simulink model "simulation"  (R2015a)
settings: Solver=ode45  StartTime=0.0  StopTime=10.0  RelTol=1e-3
libraries: powerlib x63
settings Model: Creator=Syed_Sharjeel  LastModifiedBy=Syed_Sharjeel

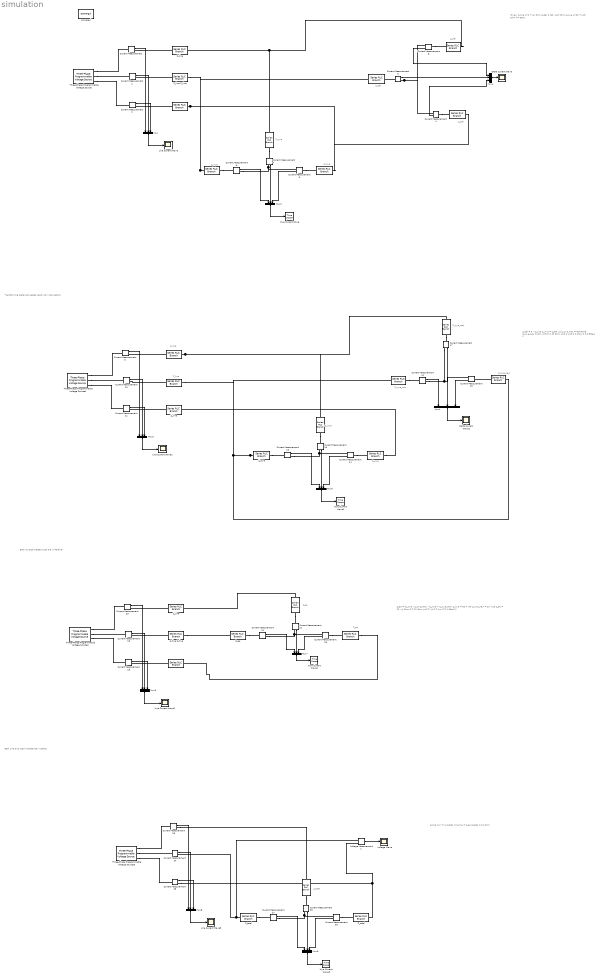
== system simulation ==
  note: Given:
      | Z_line = (2 + j4) Ohm
      | Z_del = (60 - j45) Ohm
      | Z_wye = (30 + j40) Ohm
      | f = 60Hz
  note: Z_total
  note: Z_eq
  note: Z_eq
  note: Z_line
  note: Z_line
  note: Z_wye
  note: Z_wye
  note: Z_wye
  note: Z_del
  note: Z_del
  note: Z_del
  note: Z_wye_new
  note: Z_wye_new
  note: Z_wye_new
  note: Z_wye
  note: Z_wye
  note: Z_line = 2 + j4
      | Z_total = Z_line + Z_eq
      | Z_total = 24 Ohm
  note: Both Line and Load Impedance in Series
  note: Z_eq = (Z_wye * Z_wye_new) / (Z_wye + Z_wye_new)
      | Z_wye = 30 + j40
      | Z_wye_new = 20 - j15
      | Z_eq = 22 - j4 Ohm
      | R = 22 Ohm
      | -jwC = -j4
      | C = 4/w
      | C = 1.06e-2 F
  note: Both Wye-Connected Load are in Parallel
  note: Z_del = 3 * Z_wye
      | Z_wye = Z_del / 3
      | Z_wye_new = (60-j45)/3
      | Z_wye_new = (20 - j15)
      | R = 20 Ohm
      | -jwC = -j15
      | C = 15/w
      | C = 3.98e-2 F
  note: Transforming Delta Connected Load into Y-Connection
   {,,,,} (5 alike) : powerlib/Elements/Series RLC Branch  LConnTagsString=__new0  RConnTagsString=__new0  BranchType=RL  Resistance=40  Inductance=0.66  SetiL0=off  InitialCurrent=0  Capacitance=1e-6  Setx0=off  InitialVoltage=0  Measurements=None
  " " : powerlib/Elements/Series RLC Branch  LConnTagsString=__new0  RConnTagsString=__new0  BranchType=RC  Resistance=60  Inductance=1e-3  SetiL0=off  InitialCurrent=0  Capacitance=3.703e-4  Setx0=off  InitialVoltage=0  Measurements=None
  " " : powerlib/Elements/Series RLC Branch  LConnTagsString=__new0  RConnTagsString=__new0  BranchType=RC  Resistance=20  Inductance=1e-3  SetiL0=off  InitialCurrent=0  Capacitance=3.98e-2  Setx0=off  InitialVoltage=0  Measurements=None
  " " : powerlib/Elements/Series RLC Branch  LConnTagsString=__new0  RConnTagsString=__new0  BranchType=RC  Resistance=60  Inductance=1e-3  SetiL0=off  InitialCurrent=0  Capacitance=3.703e-4  Setx0=off  InitialVoltage=0  Measurements=None
  " " : powerlib/Elements/Series RLC Branch  LConnTagsString=__new0  RConnTagsString=__new0  BranchType=RC  Resistance=20  Inductance=1e-3  SetiL0=off  InitialCurrent=0  Capacitance=3.98e-2  Setx0=off  InitialVoltage=0  Measurements=None
  " " : powerlib/Elements/Series RLC Branch  LConnTagsString=__new0  RConnTagsString=__new0  BranchType=RC  Resistance=20  Inductance=1e-3  SetiL0=off  InitialCurrent=0  Capacitance=3.98e-2  Setx0=off  InitialVoltage=0  Measurements=None
  " " : powerlib/Elements/Series RLC Branch  LConnTagsString=__new0  RConnTagsString=__new0  BranchType=RC  Resistance=60  Inductance=1e-3  SetiL0=off  InitialCurrent=0  Capacitance=3.703e-4  Setx0=off  InitialVoltage=0  Measurements=None
  " " : powerlib/Elements/Series RLC Branch  LConnTagsString=__new0  RConnTagsString=__new0  BranchType=R  Resistance=24  Inductance=0.66  SetiL0=off  InitialCurrent=0  Capacitance=1.06e-2  Setx0=off  InitialVoltage=0  Measurements=None
   {,,,} (4 alike) : powerlib/Elements/Series RLC Branch  LConnTagsString=__new0  RConnTagsString=__new0  BranchType=RL  Resistance=2  Inductance=0.066  SetiL0=off  InitialCurrent=0  Capacitance=1e-6  Setx0=off  InitialVoltage=0  Measurements=None
  " " : powerlib/Elements/Series RLC Branch  LConnTagsString=__new0  RConnTagsString=__new0  BranchType=RC  Resistance=20  Inductance=0.66  SetiL0=off  InitialCurrent=0  Capacitance=1.06e-2  Setx0=off  InitialVoltage=0  Measurements=None
  " " : powerlib/Elements/Series RLC Branch  LConnTagsString=__new0  RConnTagsString=__new0  BranchType=RC  Resistance=20  Inductance=0.66  SetiL0=off  InitialCurrent=0  Capacitance=1.06e-2  Setx0=off  InitialVoltage=0  Measurements=None
  " Z_eq " : powerlib/Elements/Series RLC Branch  LConnTagsString=__new0  RConnTagsString=__new0  BranchType=RC  Resistance=20  Inductance=0.66  SetiL0=off  InitialCurrent=0  Capacitance=1.06e-2  Setx0=off  InitialVoltage=0  Measurements=None
  " Z_line Z_line " : powerlib/Elements/Series RLC Branch  LConnTagsString=__new0  RConnTagsString=__new0  BranchType=RL  Resistance=2  Inductance=0.066  SetiL0=off  InitialCurrent=0  Capacitance=1e-6  Setx0=off  InitialVoltage=0  Measurements=None
  Current Measurement{,1..29} (30 alike) : powerlib/Measurements/Current Measurement  PhasorSimulation=off  OutputType=Complex  PSBequivalent=0
  Delta Current Wave : Scope
      settings: TimeRange=0.05  YMin=-0.09  YMax=0.12
  Delta Current Wave1 : Scope
      settings: TimeRange=0.05  YMin=-0.09  YMax=0.12  SaveName=ScopeData2
  Line Current Wave{,1..3} (4 alike) : Scope
      Line Current Wave settings: YMin=-0.025  YMax=0.025  SaveName=ScopeData4
      Line Current Wave1 settings: YMin=-0.025  YMax=0.025  SaveName=ScopeData3
      Line Current Wave2 settings: YMin=-0.025  YMax=0.025  SaveName=ScopeData5
      Line Current Wave3 settings: YMin=-0.025  YMax=0.025  SaveName=ScopeData7
  Mux{,1..9} (10 alike) : Mux  Inputs=3
  Three-Phase Programmable Voltage Source{,1..3} (4 alike) : powerlib/Electrical Sources/Three-Phase Programmable Voltage Source  PositiveSequence="[207.85  0 60]"  VariationEntity=None  VariationType=Table of time-amplitude pairs  VariationTypeAlt=Step  VariationStep=0.5  VariationRate=10  VariationMagnitude=0.3  VariationFrequency=2  VariationTiming=[1 2]  VariationPhaseA=off  Amplitudes=[1 0.8 1.2 1.0]  TimeValues=[0 0.1 0.15 0.2]  HarmonicGeneration=off  HarmonicA=[3 0.2 -25 0]  HarmonicB=[2 0.15 35 2]  Timing="[0.05  3]"  BusType=swing  Pref=0  Qref=0  Qmin=-inf  Qmax=inf
  Voltage Measurement1 : powerlib/Measurements/Voltage Measurement  PhasorSimulation=off  OutputType=Complex  PSBequivalent=0
  Voltage Wave : Scope
      settings: TimeRange=0.05  YMin=-300  YMax=300  SaveName=ScopeData11
  Wye Current Wave{,1..3} (4 alike) : TimeScope
  "Z_line " : powerlib/Elements/Series RLC Branch  LConnTagsString=__new0  RConnTagsString=__new0  BranchType=RL  Resistance=2  Inductance=0.066  SetiL0=off  InitialCurrent=0  Capacitance=1e-6  Setx0=off  InitialVoltage=0  Measurements=None
  "Z_line Z_line " : powerlib/Elements/Series RLC Branch  LConnTagsString=__new0  RConnTagsString=__new0  BranchType=RL  Resistance=2  Inductance=0.066  SetiL0=off  InitialCurrent=0  Capacitance=1e-6  Setx0=off  InitialVoltage=0  Measurements=None
  "Z_line " : powerlib/Elements/Series RLC Branch  LConnTagsString=__new0  RConnTagsString=__new0  BranchType=RL  Resistance=2  Inductance=0.066  SetiL0=off  InitialCurrent=0  Capacitance=1e-6  Setx0=off  InitialVoltage=0  Measurements=None
  "Z_line " : powerlib/Elements/Series RLC Branch  LConnTagsString=__new0  RConnTagsString=__new0  BranchType=RL  Resistance=2  Inductance=0.066  SetiL0=off  InitialCurrent=0  Capacitance=1e-6  Setx0=off  InitialVoltage=0  Measurements=None
  "Z_total " : powerlib/Elements/Series RLC Branch  LConnTagsString=__new0  RConnTagsString=__new0  BranchType=R  Resistance=24  Inductance=0.66  SetiL0=off  InitialCurrent=0  Capacitance=1.06e-2  Setx0=off  InitialVoltage=0  Measurements=None
  "Z_total " : powerlib/Elements/Series RLC Branch  LConnTagsString=__new0  RConnTagsString=__new0  BranchType=R  Resistance=24  Inductance=0.66  SetiL0=off  InitialCurrent=0  Capacitance=1.06e-2  Setx0=off  InitialVoltage=0  Measurements=None
  Z_wye : powerlib/Elements/Series RLC Branch  LConnTagsString=__new0  RConnTagsString=__new0  BranchType=RL  Resistance=40  Inductance=0.66  SetiL0=off  InitialCurrent=0  Capacitance=1e-6  Setx0=off  InitialVoltage=0  Measurements=None
  powergui : powerlib/powergui  Priority=1  SimulationMode=Discrete  SolverType=Tustin/Backward Euler (TBE)  SampleTime=5e-5  frequency=60  SPID=off  DisableSnubberDevices=off  DisableRonSwitches=off  DisableVfSwitches=off  SwTol=0  DisplayEquations=off  Interpol=off  methode=off  Ts=100  FunctionMessages=off  echomessages=off  HookPort=off  EnableUseOfTLC=off  x0status=blocks  frequencyindice=60  Pbase=100e6  ErrMax=1e-4  Iterations=50  UnitsV=kV  UnitsW=MW  buscounter=0  RestoreLinks=warning  ResistiveCurrentMeasurement=off  Frange=[0:2:500]  Ylog=off  Xlog=on  ShowGrid=off  save=off  variable=ZData  structure=0  ZoomFFT=off  StartTime=0.0  cycles=1  DisplayStyle=1  fundamental=60  FreqAxis=off  MaxFrequency=1000  frequencyindicesteady=1  RmsSteady=1  display=off
  wires:
  Current Measurement/1 -> Mux/1
  Current Measurement1/1 -> Mux/2
  Current Measurement2/1 -> Mux/3
  Mux/1 -> Line Current Wave/1
  Mux1/1 -> Delta Current Wave/1
  Current Measurement6/1 -> Mux2/1
  Current Measurement7/1 -> Mux2/2
  Current Measurement5/1 -> Mux2/3
  Mux2/1 -> Wye Current Wave/1
  Current Measurement8/1 -> Mux1/1
  Current Measurement3/1 -> Mux1/2
  Current Measurement4/1 -> Mux1/3
  Current Measurement9/1 -> Mux3/1
  Current Measurement10/1 -> Mux3/2
  Current Measurement11/1 -> Mux3/3
  Mux3/1 -> Line Current Wave1/1
  Current Measurement15/1 -> Mux5/1
  Current Measurement16/1 -> Mux5/2
  Current Measurement14/1 -> Mux5/3
  Mux5/1 -> Wye Current Wave1/1
  Current Measurement12/1 -> Mux4/1
  Current Measurement17/1 -> Mux4/2
  Current Measurement13/1 -> Mux4/3
  Mux4/1 -> Delta Current Wave1/1
  Current Measurement23/1 -> Mux6/1
  Current Measurement18/1 -> Mux6/2
  Current Measurement19/1 -> Mux6/3
  Mux6/1 -> Line Current Wave2/1
  Current Measurement21/1 -> Mux7/1
  Current Measurement22/1 -> Mux7/2
  Current Measurement20/1 -> Mux7/3
  Mux7/1 -> Wye Current Wave2/1
  Current Measurement29/1 -> Mux8/1
  Current Measurement24/1 -> Mux8/2
  Current Measurement25/1 -> Mux8/3
  Mux8/1 -> Line Current Wave3/1
  Current Measurement27/1 -> Mux9/1
  Current Measurement28/1 -> Mux9/2
  Current Measurement26/1 -> Mux9/3
  Mux9/1 -> Wye Current Wave3/1
  Voltage Measurement1/1 -> Voltage Wave/1
  connections:
  " "/RConn1 -- " "/LConn1
  " "/LConn1 -- "Z_line Z_line "/RConn1
  Current Measurement7/RConn1 -- Current Measurement6/RConn1 -- Current Measurement5/RConn1
  " "/LConn1 -- "Z_line "/RConn1
  Current Measurement3/RConn1 -- Current Measurement4/RConn1 -- Current Measurement8/RConn1
  Z_wye/LConn1 -- " "/LConn1 -- " "/RConn1
  Current Measurement14/RConn1 -- Current Measurement16/RConn1 -- Current Measurement15/RConn1
  " "/RConn1 -- " "/LConn1
  Current Measurement17/RConn1 -- Current Measurement12/RConn1 -- Current Measurement13/RConn1
  Current Measurement20/RConn1 -- Current Measurement22/RConn1 -- Current Measurement21/RConn1
  Current Measurement28/RConn1 -- Current Measurement27/RConn1 -- Current Measurement26/RConn1
  "Z_total "/LConn1 -- Voltage Measurement1/LConn1 -- Current Measurement24/RConn1
  Voltage Measurement1/LConn2 -- "Z_total "/LConn1 -- Current Measurement25/RConn1
  Three-Phase Programmable Voltage Source/RConn3 -- Current Measurement2/LConn1
  Current Measurement3/LConn1 -- " "/RConn1
  " "/RConn1 -- Current Measurement6/LConn1
  "Z_line "/LConn1 -- Current Measurement/RConn1
  Current Measurement5/LConn1 -- " "/RConn1
  " "/LConn1 -- Current Measurement2/RConn1
  " "/RConn1 -- Current Measurement7/LConn1
  Current Measurement8/LConn1 -- " "/RConn1
  Current Measurement4/LConn1 -- " "/RConn1
  Three-Phase Programmable Voltage Source/RConn1 -- Current Measurement/LConn1
  Three-Phase Programmable Voltage Source/RConn2 -- Current Measurement1/LConn1
  " "/LConn1 -- "Z_line "/RConn1
  "Z_line Z_line "/LConn1 -- Current Measurement1/RConn1
  Three-Phase Programmable Voltage Source2/RConn1 -- Current Measurement23/LConn1
  "Z_line "/LConn1 -- Current Measurement11/RConn1
  Three-Phase Programmable Voltage Source1/RConn3 -- Current Measurement11/LConn1
  Current Measurement14/LConn1 -- " "/RConn1
  " "/RConn1 -- Current Measurement13/LConn1
  " "/LConn1 -- Current Measurement10/RConn1
  " "/RConn1 -- Current Measurement16/LConn1
  Three-Phase Programmable Voltage Source1/RConn2 -- Current Measurement10/LConn1
  " "/RConn1 -- Current Measurement12/LConn1
  Three-Phase Programmable Voltage Source1/RConn1 -- Current Measurement9/LConn1
  " "/LConn1 -- Current Measurement9/RConn1
  Z_wye/RConn1 -- Current Measurement15/LConn1
  " "/RConn1 -- Current Measurement17/LConn1
  " Z_line Z_line "/LConn1 -- Current Measurement18/RConn1
  Three-Phase Programmable Voltage Source2/RConn2 -- Current Measurement18/LConn1
  Current Measurement29/RConn1 -- " "/LConn1
  " "/LConn1 -- " "/RConn1
  Three-Phase Programmable Voltage Source2/RConn3 -- Current Measurement19/LConn1
  Three-Phase Programmable Voltage Source3/RConn1 -- Current Measurement29/LConn1
  "Z_total "/RConn1 -- Current Measurement27/LConn1
  Three-Phase Programmable Voltage Source3/RConn2 -- Current Measurement24/LConn1
  " "/RConn1 -- Current Measurement28/LConn1
  Three-Phase Programmable Voltage Source3/RConn3 -- Current Measurement25/LConn1
  " "/LConn1 -- Current Measurement19/RConn1
  " Z_line Z_line "/RConn1 -- " Z_eq "/LConn1
  Current Measurement20/LConn1 -- " "/RConn1
  " "/RConn1 -- Current Measurement22/LConn1
  Current Measurement26/LConn1 -- "Z_total "/RConn1
  " Z_eq "/RConn1 -- Current Measurement21/LConn1
  "Z_line "/LConn1 -- Current Measurement23/RConn1
  " "/LConn1 -- "Z_line "/RConn1
